simulink library "nist_library"  (R2012b)
settings: Solver=VariableStepDiscrete  StartTime=0  StopTime=1000  RelTol=1e-3
undefined symbols (not defined in the file or in its folder): A, B, C, D, sfp, xlipgetpartsetting
libraries: xbsIndex_r4 x385, xps_library x44, nist_library x4, casper_library_misc x4, casper_library_delays x1
(part 2 of 11)

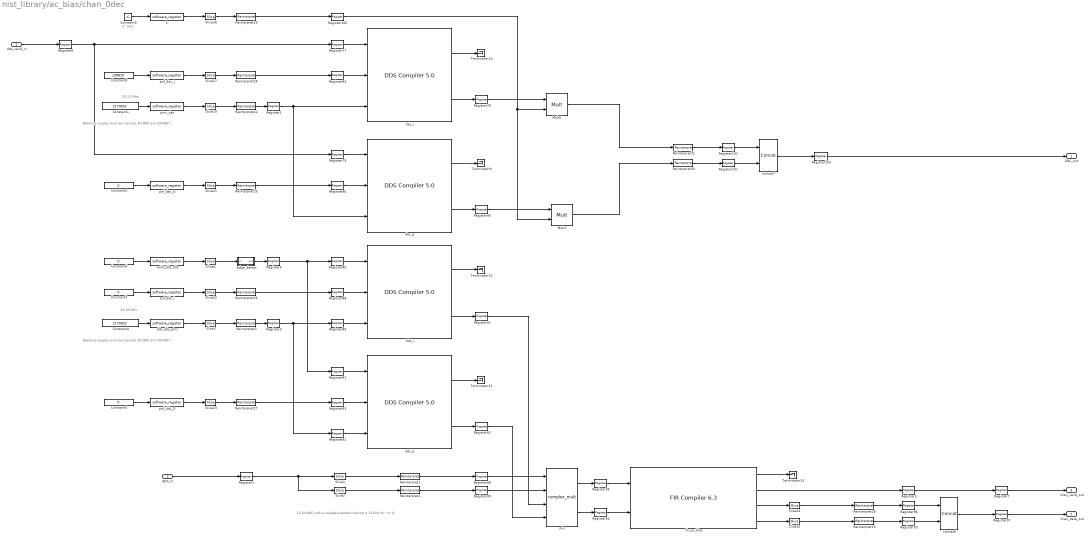
== system nist_library/ac_bias/chan_0dec ==
  note: 33.10 MHz
  note: Absolute angles must be inputed.
      | All DDS are COSINE().
  note: 33.10 MHz
  note: Absolute angles must be inputed.
      | All DDS are COSINE().
  note: 12 bit ADC with a coadded sample making it
      | 13 bits for I or Q
  dds_valid_in : Inport
  ADC_In : Inport  Port=2
  Concat6 : xbsIndex_r4/Concat  num_inputs=2  dbl_ovrd=off  block_type=concat
  Concat7 : xbsIndex_r4/Concat  num_inputs=2  dbl_ovrd=off  block_type=concat
  Constant1 : Constant  Value=2170652
  Constant{2..3,5..6} (4 alike) : Constant  Value=0
  Constant4 : Constant  Value=2170652
  Constant8 : Constant  Value=139810
  Constant9 : Constant  Value=2^15-1
  Mult0 : xbsIndex_r4/Mult  precision=User Defined  arith_type="Signed  (2's comp)"  n_bits=16  bin_pt=15  quantization=Truncate  overflow=Wrap  en=off  latency=4  dbl_ovrd=off  use_behavioral_HDL=off  opt=Area  use_embedded=off  optimum_pipeline=on  pipeline=on  use_rpm=on  placement_style=Triangular  block_type=mult
  Mult1 : xbsIndex_r4/Mult  precision=User Defined  arith_type="Signed  (2's comp)"  n_bits=16  bin_pt=15  quantization=Truncate  overflow=Wrap  en=off  latency=4  dbl_ovrd=off  use_behavioral_HDL=off  opt=Area  use_embedded=off  optimum_pipeline=on  pipeline=on  use_rpm=on  placement_style=Triangular  block_type=mult
  Register{1..7,77..84,86,88..103} (32 alike) : xbsIndex_r4/Register  init=0  rst=off  en=off  dbl_ovrd=off  block_type=register
  Reinterpret1 : xbsIndex_r4/Reinterpret  force_arith_type=on  arith_type="Signed  (2's comp)"  force_bin_pt=on  bin_pt=11  block_type=reinterpret
      settings: block_version=10.1.3
  Reinterpret2 : xbsIndex_r4/Reinterpret  force_arith_type=on  arith_type="Signed  (2's comp)"  force_bin_pt=on  bin_pt=11  block_type=reinterpret
      settings: block_version=10.1.3
  Reinterpret{3,22,24..27} (6 alike) : xbsIndex_r4/Reinterpret  force_arith_type=on  arith_type="Signed  (2's comp)"  force_bin_pt=on  bin_pt=24  block_type=reinterpret
      settings: block_version=10.1.3
  Reinterpret{23,28,30..31} (4 alike) : xbsIndex_r4/Reinterpret  force_arith_type=on  arith_type=Unsigned  force_bin_pt=on  bin_pt=0  block_type=reinterpret
      settings: block_version=10.1.3
  Reinterpret29 : xbsIndex_r4/Reinterpret  force_arith_type=on  arith_type="Signed  (2's comp)"  force_bin_pt=on  bin_pt=15  block_type=reinterpret
      settings: block_version=10.1.3
  Slice1 : xbsIndex_r4/Slice  nbits=13  boolean_output=off  mode=Lower Bit Location + Width  bit1=2  base1=Binary Point of Input  bit0=13  base0=LSB of Input  dbl_ovrd=off  block_type=slice
      settings: block_version=10.1.3
  Slice2 : xbsIndex_r4/Slice  nbits=13  boolean_output=off  mode=Lower Bit Location + Width  bit1=2  base1=Binary Point of Input  bit0=0  base0=LSB of Input  dbl_ovrd=off  block_type=slice
      settings: block_version=10.1.3
  Slice{3,21..23,27,29} (6 alike) : xbsIndex_r4/Slice  nbits=24  boolean_output=off  mode=Lower Bit Location + Width  bit1=0  base1=MSB of Input  bit0=0  base0=LSB of Input  dbl_ovrd=off  block_type=slice
      settings: block_version=10.1.3
  Slice24 : xbsIndex_r4/Slice  nbits=32  boolean_output=off  mode=Two Bit Locations  bit1=2  base1=Binary Point of Input  bit0=-18  base0=Binary Point of Input  dbl_ovrd=off  block_type=slice
      settings: block_version=10.1.3
  Slice25 : xbsIndex_r4/Slice  nbits=32  boolean_output=off  mode=Two Bit Locations  bit1=2  base1=Binary Point of Input  bit0=-18  base0=Binary Point of Input  dbl_ovrd=off  block_type=slice
      settings: block_version=10.1.3
  Slice26 : xbsIndex_r4/Slice  nbits=16  boolean_output=off  mode=Lower Bit Location + Width  bit1=0  base1=MSB of Input  bit0=0  base0=LSB of Input  dbl_ovrd=off  block_type=slice
      settings: block_version=10.1.3
  Slice4 : xbsIndex_r4/Slice  nbits=24  boolean_output=on  mode=Lower Bit Location + Width  bit1=0  base1=MSB of Input  bit0=0  base0=LSB of Input  dbl_ovrd=off  block_type=slice
      settings: block_version=10.1.3
  Terminator{9..11,13..14} (5 alike) : Terminator
  dac_I : xbsIndex_r4/DDS Compiler 5.0   partspresent=Phase_Generator_and_SIN_COS_LUT  dds_clock_rate=256  channels=1  parameter_entry=Hardware_Parameters  spurious_free_dynamic_range=36  frequency_resolution=0.4  noise_shaping=None  phase_width=24  output_width=16  output_selection=Cosine  negative_sine=off  negative_cosine=off  amplitude_mode=Full_Range  memory_type=Block_ROM  optimization_goal=Speed  dsp48_use=Minimal  latency_configuration=Auto  latency=4  has_phase_out=off  has_aclken=off  has_aresetn=off  explicit_period=off  period=1  data_has_tlast=Not_Required  has_tready=off  s_phase_has_tuser=Not_Required  m_data_has_tuser=Not_Required  m_phase_has_tuser=Not_Required  s_phase_tuser_width=1  s_config_sync_mode=On_Vector  phase_increment=Programmable  output_frequency1=0  output_frequency2=0  output_frequency3=0  output_frequency4=0  output_frequency5=0  output_frequency6=0  output_frequency7=0  output_frequency8=0  output_frequency9=0  output_frequency10=0  output_frequency11=0  output_frequency12=0  output_frequency13=0  output_frequency14=0  output_frequency15=0  output_frequency16=0  pinc1='1101000110110'  pinc2='0'  pinc3='0'  pinc4='0'  pinc5='0'  pinc6='0'  pinc7='0'  pinc8='0'  pinc9='0'  pinc10='0'  pinc11='0'  pinc12='0'  pinc13='0'  pinc14='0'  pinc15='0'  pinc16='0'  phase_offset=Programmable  phase_offset_angles1=0  phase_offset_angles2=0  phase_offset_angles3=0  phase_offset_angles4=0  phase_offset_angles5=0  phase_offset_angles6=0  phase_offset_angles7=0  phase_offset_angles8=0  phase_offset_angles9=0  phase_offset_angles10=0  phase_offset_angles11=0  phase_offset_angles12=0  phase_offset_angles13=0  phase_offset_angles14=0  phase_offset_angles15=0  phase_offset_angles16=0  poff1='0'  poff2='0'  poff3='0'  poff4='0'  poff5='0'  poff6='0'  poff7='0'  poff8='0'  poff9='0'  poff10='0'  poff11='0'  poff12='0'  poff13='0'  poff14='0'  poff15='0'  poff16='0'  trim_axipin_name=on  por_mode=false  gui_behaviour=Sysgen  ip_name=DDS Compiler  ip_version=5.0  dsptool_ready=true  wrapper_available=true  port_translation_map={ 'aclken' => 'en', 'aresetn' => 'rst' }  ipcore_xco_need_fpga_part=true  ipcore_fpga_part=xlipgetpartsetting(gcb, {'virtex6', 'xc6vlx75t', '-3', 'ff784'})  ipcore_usecache=true  ipcore_useipmodelcache=true  ipcore_verbose=false  block_type=dds_compiler_v5_0
  dac_q : xbsIndex_r4/DDS Compiler 5.0   partspresent=Phase_Generator_and_SIN_COS_LUT  dds_clock_rate=256  channels=1  parameter_entry=Hardware_Parameters  spurious_free_dynamic_range=36  frequency_resolution=0.4  noise_shaping=None  phase_width=24  output_width=16  output_selection=Sine  negative_sine=off  negative_cosine=off  amplitude_mode=Full_Range  memory_type=Block_ROM  optimization_goal=Speed  dsp48_use=Minimal  latency_configuration=Auto  latency=8  has_phase_out=off  has_aclken=off  has_aresetn=off  explicit_period=off  period=1  data_has_tlast=Not_Required  has_tready=off  s_phase_has_tuser=Not_Required  m_data_has_tuser=Not_Required  m_phase_has_tuser=Not_Required  s_phase_tuser_width=1  s_config_sync_mode=On_Vector  phase_increment=Programmable  output_frequency1=0  output_frequency2=0  output_frequency3=0  output_frequency4=0  output_frequency5=0  output_frequency6=0  output_frequency7=0  output_frequency8=0  output_frequency9=0  output_frequency10=0  output_frequency11=0  output_frequency12=0  output_frequency13=0  output_frequency14=0  output_frequency15=0  output_frequency16=0  pinc1='1101000110110'  pinc2='0'  pinc3='0'  pinc4='0'  pinc5='0'  pinc6='0'  pinc7='0'  pinc8='0'  pinc9='0'  pinc10='0'  pinc11='0'  pinc12='0'  pinc13='0'  pinc14='0'  pinc15='0'  pinc16='0'  phase_offset=Programmable  phase_offset_angles1=0  phase_offset_angles2=0  phase_offset_angles3=0  phase_offset_angles4=0  phase_offset_angles5=0  phase_offset_angles6=0  phase_offset_angles7=0  phase_offset_angles8=0  phase_offset_angles9=0  phase_offset_angles10=0  phase_offset_angles11=0  phase_offset_angles12=0  phase_offset_angles13=0  phase_offset_angles14=0  phase_offset_angles15=0  phase_offset_angles16=0  poff1='0'  poff2='0'  poff3='0'  poff4='0'  poff5='0'  poff6='0'  poff7='0'  poff8='0'  poff9='0'  poff10='0'  poff11='0'  poff12='0'  poff13='0'  poff14='0'  poff15='0'  poff16='0'  trim_axipin_name=on  por_mode=false  gui_behaviour=Sysgen  ip_name=DDS Compiler  ip_version=5.0  dsptool_ready=true  wrapper_available=true  port_translation_map={ 'aclken' => 'en', 'aresetn' => 'rst' }  ipcore_xco_need_fpga_part=true  ipcore_fpga_part=xlipgetpartsetting(gcb, {'virtex6', 'xc6vlx75t', '-3', 'ff784'})  ipcore_usecache=true  ipcore_useipmodelcache=true  ipcore_verbose=false  block_type=dds_compiler_v5_0
  ddc_I : xbsIndex_r4/DDS Compiler 5.0   partspresent=Phase_Generator_and_SIN_COS_LUT  dds_clock_rate=256  channels=1  parameter_entry=Hardware_Parameters  spurious_free_dynamic_range=36  frequency_resolution=0.4  noise_shaping=None  phase_width=24  output_width=13  output_selection=Cosine  negative_sine=off  negative_cosine=off  amplitude_mode=Full_Range  memory_type=Block_ROM  optimization_goal=Speed  dsp48_use=Minimal  latency_configuration=Auto  latency=4  has_phase_out=off  has_aclken=off  has_aresetn=off  explicit_period=off  period=1  data_has_tlast=Not_Required  has_tready=off  s_phase_has_tuser=Not_Required  m_data_has_tuser=Not_Required  m_phase_has_tuser=Not_Required  s_phase_tuser_width=1  s_config_sync_mode=On_Vector  phase_increment=Programmable  output_frequency1=0  output_frequency2=0  output_frequency3=0  output_frequency4=0  output_frequency5=0  output_frequency6=0  output_frequency7=0  output_frequency8=0  output_frequency9=0  output_frequency10=0  output_frequency11=0  output_frequency12=0  output_frequency13=0  output_frequency14=0  output_frequency15=0  output_frequency16=0  pinc1='1101000110110'  pinc2='0'  pinc3='0'  pinc4='0'  pinc5='0'  pinc6='0'  pinc7='0'  pinc8='0'  pinc9='0'  pinc10='0'  pinc11='0'  pinc12='0'  pinc13='0'  pinc14='0'  pinc15='0'  pinc16='0'  phase_offset=Programmable  phase_offset_angles1=0  phase_offset_angles2=0  phase_offset_angles3=0  phase_offset_angles4=0  phase_offset_angles5=0  phase_offset_angles6=0  phase_offset_angles7=0  phase_offset_angles8=0  phase_offset_angles9=0  phase_offset_angles10=0  phase_offset_angles11=0  phase_offset_angles12=0  phase_offset_angles13=0  phase_offset_angles14=0  phase_offset_angles15=0  phase_offset_angles16=0  poff1='0'  poff2='0'  poff3='0'  poff4='0'  poff5='0'  poff6='0'  poff7='0'  poff8='0'  poff9='0'  poff10='0'  poff11='0'  poff12='0'  poff13='0'  poff14='0'  poff15='0'  poff16='0'  trim_axipin_name=on  por_mode=false  gui_behaviour=Sysgen  ip_name=DDS Compiler  ip_version=5.0  dsptool_ready=true  wrapper_available=true  port_translation_map={ 'aclken' => 'en', 'aresetn' => 'rst' }  ipcore_xco_need_fpga_part=true  ipcore_fpga_part=xlipgetpartsetting(gcb, {'virtex6', 'xc6vlx75t', '-3', 'ff784'})  ipcore_usecache=true  ipcore_useipmodelcache=true  ipcore_verbose=false  block_type=dds_compiler_v5_0
  ddc_q : xbsIndex_r4/DDS Compiler 5.0   partspresent=Phase_Generator_and_SIN_COS_LUT  dds_clock_rate=256  channels=1  parameter_entry=Hardware_Parameters  spurious_free_dynamic_range=36  frequency_resolution=0.4  noise_shaping=None  phase_width=24  output_width=13  output_selection=Sine  negative_sine=off  negative_cosine=off  amplitude_mode=Full_Range  memory_type=Block_ROM  optimization_goal=Speed  dsp48_use=Minimal  latency_configuration=Auto  latency=8  has_phase_out=off  has_aclken=off  has_aresetn=off  explicit_period=off  period=1  data_has_tlast=Not_Required  has_tready=off  s_phase_has_tuser=Not_Required  m_data_has_tuser=Not_Required  m_phase_has_tuser=Not_Required  s_phase_tuser_width=1  s_config_sync_mode=On_Vector  phase_increment=Programmable  output_frequency1=0  output_frequency2=0  output_frequency3=0  output_frequency4=0  output_frequency5=0  output_frequency6=0  output_frequency7=0  output_frequency8=0  output_frequency9=0  output_frequency10=0  output_frequency11=0  output_frequency12=0  output_frequency13=0  output_frequency14=0  output_frequency15=0  output_frequency16=0  pinc1='1101000110110'  pinc2='0'  pinc3='0'  pinc4='0'  pinc5='0'  pinc6='0'  pinc7='0'  pinc8='0'  pinc9='0'  pinc10='0'  pinc11='0'  pinc12='0'  pinc13='0'  pinc14='0'  pinc15='0'  pinc16='0'  phase_offset=Programmable  phase_offset_angles1=0  phase_offset_angles2=0  phase_offset_angles3=0  phase_offset_angles4=0  phase_offset_angles5=0  phase_offset_angles6=0  phase_offset_angles7=0  phase_offset_angles8=0  phase_offset_angles9=0  phase_offset_angles10=0  phase_offset_angles11=0  phase_offset_angles12=0  phase_offset_angles13=0  phase_offset_angles14=0  phase_offset_angles15=0  phase_offset_angles16=0  poff1='0'  poff2='0'  poff3='0'  poff4='0'  poff5='0'  poff6='0'  poff7='0'  poff8='0'  poff9='0'  poff10='0'  poff11='0'  poff12='0'  poff13='0'  poff14='0'  poff15='0'  poff16='0'  trim_axipin_name=on  por_mode=false  gui_behaviour=Sysgen  ip_name=DDS Compiler  ip_version=5.0  dsptool_ready=true  wrapper_available=true  port_translation_map={ 'aclken' => 'en', 'aresetn' => 'rst' }  ipcore_xco_need_fpga_part=true  ipcore_fpga_part=xlipgetpartsetting(gcb, {'virtex6', 'xc6vlx75t', '-3', 'ff784'})  ipcore_usecache=true  ipcore_useipmodelcache=true  ipcore_verbose=false  block_type=dds_compiler_v5_0
  dds_ddc_pinc : xps_library/software_register  Tag=xps:sw_reg  mode=one value  io_dir=From Processor  io_delay=0  sample_period=1  names=reg  bitwidths=32  arith_types=0  bin_pts=0  sim_port=on  show_format=off
      settings: AttributesFormatString=1input
  edge_detect : Subsystem  AncestorBlock=casper_library_misc/edge_detect  mask(edge_detect){edge=Rising, polarity=Active High, x_in=[0 0.08 0.08 0.16 0.16 0.24 0.24 0.32 0.32 0.4], y_in=[-1 -1  1  1  1  1  1  1  1  1], x_out=[0.6 0.68 0.68 0.76 0.76 0.84 0.84 0.92 0.92 1], y_out=[-1 -1  1  1 -1 -1 -1 -1 -1 -1]}
      mask prompts: edge "Edge Type"; polarity "Output Polarity"; x_in "Input X Positions"; y_in "Input Y Positions"; x_out "Output X Positions"; y_out "Output Y Positions"
      mask help: Output is active for one-cycle after each edge of the specified type (i.e. rising, falling or both).
      mask init: same as nist_library/ac_bias/chan/edge_detect
      settings: AttributesFormatString=|
      | rising edges
      | active high
      mask Help: Output is active for one-cycle after each edge of the specified type (i.e. rising, falling, or both).  Latency is zero.
      mask TypeOptions edge: Rising | Falling | Both
      mask TypeOptions polarity: Active High | Active Low
      mask Display:
      | plot(x_in_num,0.5+y_in_num*0.2);
      | plot(x_out_num,0.5+y_out_num*0.2);
  fir_ac_bias : xbsIndex_r4/FIR Compiler 6.3   coefficientvector=[-0.0000051764451878,0.0000745826627445,0.0001297921838022,0.0001874032893959,0.0002069390086742,0.0001661868276461,0.0000690773761229,-0.0000498999745140,-0.0001378566934410,-0.0001494152464808,-0.0000737426820472,0.0000534566516457,0.0001631966315417,0.0001883405361701,0.0001032086742222,-0.0000554836566731,-0.0002019925511815,-0.0002463508193789,-0.0001481137859129,0.0000524105583153,0.0002476389719838,0.0003189708688799,0.0002072986623486,-0.0000433125087902,-0.0002990483193093,-0.0004061365706640,-0.0002817096891831,0.0000271129031178,0.0003559545094189,0.0005087976123048,0.0003730692798155,-0.0000023723087206,-0.0004182289757719,-0.0006283441510575,-0.0004835190138798,-0.0000325469489783,0.0004856937323099,0.0007662684702860,0.0006154769248808,0.0000796164486021,-0.0005580808889874,-0.0009242247428880,-0.0007716121335212,-0.0001410015752776,0.0006350086931378,0.0011039993324493,0.0009549192219689,0.0002191539867891,-0.0007160584058988,-0.0013075266807934,-0.0011687015554378,-0.0003167990662505,0.0008007914635773,0.0015371347548913,0.0014168251716176,0.0004372635775068,-0.0008884962074707,-0.0017952386862154,-0.0017036132887631,-0.0005841367988305,0.0009785443896989,0.0020848889683874,0.0020342286514796,0.0007617264960662,-0.0010702136394660,-0.0024097893927453,-0.0024149180905617,-0.0009752647588671,0.0011626913403311,0.0027744545803019,0.0028533480821718,0.0012310737079905,-0.0012551025747609,-0.0031847282935193,-0.0033592048942565,-0.0015370858298841,0.0013465563844382,0.0036482685378070,0.0039450669725666,0.0019034710371218,-0.0014361288626481,-0.0041754398250749,-0.0046277072538667,-0.0023437115160264,0.0015228848662531,0.0047806001910473,0.0054302104189028,0.0028762154803440,-0.0016058822476575,-0.0054842390877931,-0.0063853326449652,-0.0035270741194097,0.0016842141518068,0.0063165742036384,0.0075413384085286,0.0043347523854386,-0.0017569781675854,-0.0073238906209854,-0.0089724022218468,-0.0053587076677590,0.0018233800633980,0.0085805580796381,0.0107987571293999,0.0066962769793258,-0.0018828136714446,-0.0102137734949970,-0.0132290770977612,-0.0085195863880940,0.0019340616592901,0.0124578784167174,0.0166571938566131,0.0111614947808119,-0.0019770409902282,-0.0158002995142622,-0.0219300460196766,-0.0153666051453534,0.0020110293495967,0.0214381548095281,0.0312508004544701,0.0232033548022280,-0.0020355815642907,-0.0333085181945276,-0.0527018588317399,-0.0433616484819353,0.0020504040218475,0.0763538282620906,0.1590380705037843,0.2235846111154252,0.2479446464651392,0.2235846111154252,0.1590380705037843,0.0763538282620906,0.0020504040218475,-0.0433616484819353,-0.0527018588317399,-0.0333085181945276,-0.0020355815642907,0.0232033548022280,0.0312508004544701,0.0214381548095281,0.0020110293495967,-0.0153666051453534,-0.0219300460196766,-0.0158002995142622,-0.0019770409902282,0.0111614947808119,0.0166571938566131,0.0124578784167174,0.0019340616592901,-0.0085195863880940,-0.0132290770977612,-0.0102137734949970,-0.0018828136714446,0.0066962769793258,0.0107987571293999,0.0085805580796381,0.0018233800633980,-0.0053587076677590,-0.0089724022218468,-0.0073238906209854,-0.0017569781675854,0.0043347523854386,0.0075413384085286,0.0063165742036384,0.0016842141518068,-0.0035270741194097,-0.0063853326449652,-0.0054842390877931,-0.0016058822476575,0.0028762154803440,0.0054302104189028,0.0047806001910473,0.0015228848662531,-0.0023437115160264,-0.0046277072538667,-0.0041754398250749,-0.0014361288626481,0.0019034710371218,0.0039450669725666,0.0036482685378070,0.0013465563844382,-0.0015370858298841,-0.0033592048942565,-0.0031847282935193,-0.0012551025747609,0.0012310737079905,0.0028533480821718,0.0027744545803019,0.0011626913403311,-0.0009752647588671,-0.0024149180905617,-0.0024097893927453,-0.0010702136394660,0.0007617264960662,0.0020342286514796,0.0020848889683874,0.0009785443896989,-0.0005841367988305,-0.0017036132887631,-0.0017952386862154,-0.0008884962074707,0.0004372635775068,0.0014168251716176,0.0015371347548913,0.0008007914635773 ...(+1014 chars)]  coefficient_sets=1  coefficient_reload=off  filter_type=Single_Rate  rate_change_type=Integer  interpolation_rate=1  decimation_rate=1  zero_pack_factor=1  channel_sequence=Basic  number_channels=1  pattern_list='P4-0,P4-1,P4-2,P4-3,P4-4'  number_paths=2  ratespecification=Maximum_Possible  sampleperiod=1  hardwareoversamplingrate=1  coefficient_sign=Signed  quantization=Maximize_Dynamic_Range  coefficient_width=14  bestprecision=on  coefficient_fractional_bits=15  coefficient_structure=Inferred  output_rounding_mode=Full_Precision  output_width=33  filter_architecture=Systolic_Multiply_Accumulate  optimization_goal=Area  data_buffer_type=Automatic  coefficient_buffer_type=Automatic  input_buffer_type=Not_Applicable  output_buffer_type=Not_Applicable  preference_for_other_storage=Automatic  multi_column_support=Automatic  columnconfig='48,48,33'  inter_column_pipe_length=4  data_has_tlast=Not_Required  m_data_has_tready=off  s_data_has_fifo=off  s_data_has_tuser=Not_Required  m_data_has_tuser=Not_Required  s_config_sync_mode=On_Vector  s_config_method=Single  num_reload_slots=1  has_aclken=off  has_aresetn=off  infoeditControl=ARESETn must be asserted for a minimum of 2 cycles  trim_axipin_name=on  passband_min=0.0  passband_max=0.5  stopband_min=0.5  stopband_max=1.0  filter_selection=1  gui_behaviour=Sysgen_GUI  data_sign=Signed  data_width=16  data_fractional_bits=0  data_tuser_width=1  wrapper_available=true  ip_wrap_arbitrary_binary_point=true  ip_name=FIR Compiler  ip_version=6.3  dsptool_ready=true  ipcore_usecache=true  ipcore_useipmodelcache=true  ipcore_xco_need_fpga_part=true  port_translation_map={ 'aclken' => 'en', 'aresetn' => 'rst' }  run_core_at_system_period=true  ipcore_fpga_part=xlipgetpartsetting(gcb, {'virtex6', 'xc6vlx75t', '-3', 'ff784'})  block_type=fir_compiler_v6_3
      settings: infoedit=Maximum Possible : Maximizes oversampling rate. Abstracted input handshake (no s_data_tvalid) and automatic rate propagation.<br>Hardware Oversampling Rate : Specifies oversampling rate relative to the input sample period. Abstracted input handshake (no s_data_tvalid) and automatic rate propagation.<br>Sample Period : Specifies absolute oversampling rate. No input handshake abstraction (exposes s_data_tvalid) and no rate propagation.
  k : xps_library/software_register  Tag=xps:sw_reg  mode=one value  io_dir=From Processor  io_delay=0  sample_period=1  names=reg  bitwidths=32  arith_types=0  bin_pts=0  sim_port=on  show_format=off
      settings: AttributesFormatString=1input
  mix : nist_library/utility/complex_mult
  pinc_dac : xps_library/software_register  Tag=xps:sw_reg  mode=one value  io_dir=From Processor  io_delay=0  sample_period=1  names=reg  bitwidths=32  arith_types=0  bin_pts=0  sim_port=on  show_format=off
      settings: AttributesFormatString=1input
  pof_dac_I : xps_library/software_register  Tag=xps:sw_reg  mode=one value  io_dir=From Processor  io_delay=0  sample_period=1  names=reg  bitwidths=32  arith_types=0  bin_pts=0  sim_port=on  show_format=off
      settings: AttributesFormatString=1input
  pof_dac_Q : xps_library/software_register  Tag=xps:sw_reg  mode=one value  io_dir=From Processor  io_delay=0  sample_period=1  names=reg  bitwidths=32  arith_types=0  bin_pts=0  sim_port=on  show_format=off
      settings: AttributesFormatString=1input
  pof_ddc_I : xps_library/software_register  Tag=xps:sw_reg  mode=one value  io_dir=From Processor  io_delay=0  sample_period=1  names=reg  bitwidths=32  arith_types=0  bin_pts=0  sim_port=on  show_format=off
      settings: AttributesFormatString=1input
  pof_ddc_Q : xps_library/software_register  Tag=xps:sw_reg  mode=one value  io_dir=From Processor  io_delay=0  sample_period=1  names=reg  bitwidths=32  arith_types=0  bin_pts=0  sim_port=on  show_format=off
      settings: AttributesFormatString=1input
  valid_ddc_dds : xps_library/software_register  Tag=xps:sw_reg  mode=one value  io_dir=From Processor  io_delay=0  sample_period=1  names=reg  bitwidths=32  arith_types=0  bin_pts=0  sim_port=on  show_format=off
      settings: AttributesFormatString=1input
  DAC_out : Outport
  chan_data_out : Outport  Port=2
  chan_valid_out : Outport  Port=3
  wires:
  Register7/1 -> chan_valid_out/1
  Register5/1 -> Register7/1
  Register4/1 -> Register80/1, Register81/1
  edge_detect/1(out) -> Register4/1
  Reinterpret3/1 -> Register3/1
  Slice3/1 -> Reinterpret3/1
  Slice4/1 -> edge_detect/1(in)
  valid_ddc_dds/1 -> Slice4/1
  Constant6/1 -> valid_ddc_dds/1
  dds_ddc_pinc/1 -> Slice3/1
  Constant4/1 -> dds_ddc_pinc/1
  Register92/1 -> mix/4
  Register91/1 -> mix/3
  Register3/1 -> Register89/1, Register82/1
  Register6/1 -> Register77/1, Register79/1
  Reinterpret1/1 -> Register99/1
  Reinterpret2/1 -> Register98/1
  Register2/1 -> Slice1/1, Slice2/1
  ADC_In/1 -> Register2/1
  Slice2/1 -> Reinterpret1/1
  Slice1/1 -> Reinterpret2/1
  pof_dac_Q/1 -> Slice21/1
  Constant2/1 -> pof_dac_Q/1
  Register79/1 -> dac_q/1
  pinc_dac/1 -> Slice29/1
  pof_dac_I/1 -> Slice27/1
  Constant8/1 -> pof_dac_I/1
  Register77/1 -> dac_I/1
  Slice29/1 -> Reinterpret22/1
  Slice27/1 -> Reinterpret24/1
  dac_I/1 -> Terminator14/1
  dds_valid_in/1 -> Register6/1
  Constant1/1 -> pinc_dac/1
  pof_ddc_Q/1 -> Slice23/1
  Constant5/1 -> pof_ddc_Q/1
  Slice23/1 -> Reinterpret27/1
  Reinterpret22/1 -> Register1/1
  Reinterpret25/1 -> Register86/1
  Register100/1 -> Mult0/2, Mult1/2
  Register80/1 -> ddc_I/1
  Register88/1 -> ddc_I/2
  pof_ddc_I/1 -> Slice22/1
  Concat7/1 -> Register103/1
  Reinterpret27/1 -> Register83/1
  Register89/1 -> ddc_I/3
  Register98/1 -> mix/1
  Register86/1 -> dac_q/2
  Reinterpret30/1 -> Register101/1
  Reinterpret31/1 -> Register102/1
  Register90/1 -> Mult1/1
  fir_ac_bias/3 -> Slice24/1
  Register96/1 -> Concat6/1
  Register93/1 -> Concat6/2
  fir_ac_bias/2 -> Register5/1
  Register94/1 -> fir_ac_bias/2
  Register95/1 -> fir_ac_bias/1
  Reinterpret28/1 -> Register96/1
  Reinterpret23/1 -> Register93/1
  Concat6/1 -> Register97/1
  mix/1 -> Register95/1
  mix/2 -> Register94/1
  Register97/1 -> chan_data_out/1
  Register99/1 -> mix/2
  dac_q/1 -> Terminator9/1
  Slice21/1 -> Reinterpret25/1
  Reinterpret26/1 -> Register88/1
  Register81/1 -> ddc_q/1
  Register1/1 -> dac_q/3, dac_I/3
  Register83/1 -> ddc_q/2
  Register103/1 -> DAC_out/1
  Slice22/1 -> Reinterpret26/1
  Reinterpret24/1 -> Register84/1
  ddc_q/1 -> Terminator11/1
  ddc_I/1 -> Terminator10/1
  dac_I/2 -> Register78/1
  Register84/1 -> dac_I/2
  Register82/1 -> ddc_q/3
  ddc_I/2 -> Register91/1
  Mult1/1 -> Reinterpret30/1
  dac_q/2 -> Register90/1
  Slice25/1 -> Reinterpret23/1
  Slice24/1 -> Reinterpret28/1
  fir_ac_bias/1 -> Terminator13/1
  fir_ac_bias/4 -> Slice25/1
  Constant3/1 -> pof_ddc_I/1
  ddc_q/2 -> Register92/1
  Register78/1 -> Mult0/1
  k/1 -> Slice26/1
  Slice26/1 -> Reinterpret29/1
  Constant9/1 -> k/1
  Mult0/1 -> Reinterpret31/1
  Register102/1 -> Concat7/1
  Register101/1 -> Concat7/2
  Reinterpret29/1 -> Register100/1

== system nist_library/channelized_fir/channelized_fir ==

== system nist_library/channelized_fir/channelized_symmetric_fir ==
